simulink model "camara_termicaprofwilkley_editado_0527"  (R2022a)
settings: Solver=VariableStepAuto  StartTime=0.0  StopTime=400  RelTol=1e-3
values from neighbouring files (symbols this model uses):
  Ha = Hss.A    [Camara_Termica.m]
  Hb = Hss.B    [Camara_Termica.m]
  Hc = Hss.C    [Camara_Termica.m]
  Kcurioso = [K1 K2 K3 K4]    [Camara_Termica.m]
  Kxlinha = [Kx(:,1), Kx(:,3), Kx(:,2), Kx(:,4)]    [Camara_Termica.m]
  T = conv(T,[1 alpha])    [Camara_Termica.m]
settings Model: Creator=CARLOS HOLANDA  LastModifiedBy=CARLOS HOLANDA
settings DebuggingCC: UnconnectedInputMsg=warning  UnconnectedOutputMsg=warning  UnconnectedLineMsg=warning
settings RTWCC: DLArmComputeVersion=19.05

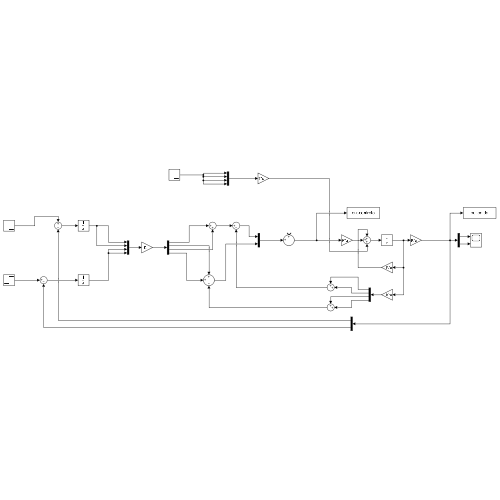
[thumbnail: Simulink's stored preview of the top-level diagram]
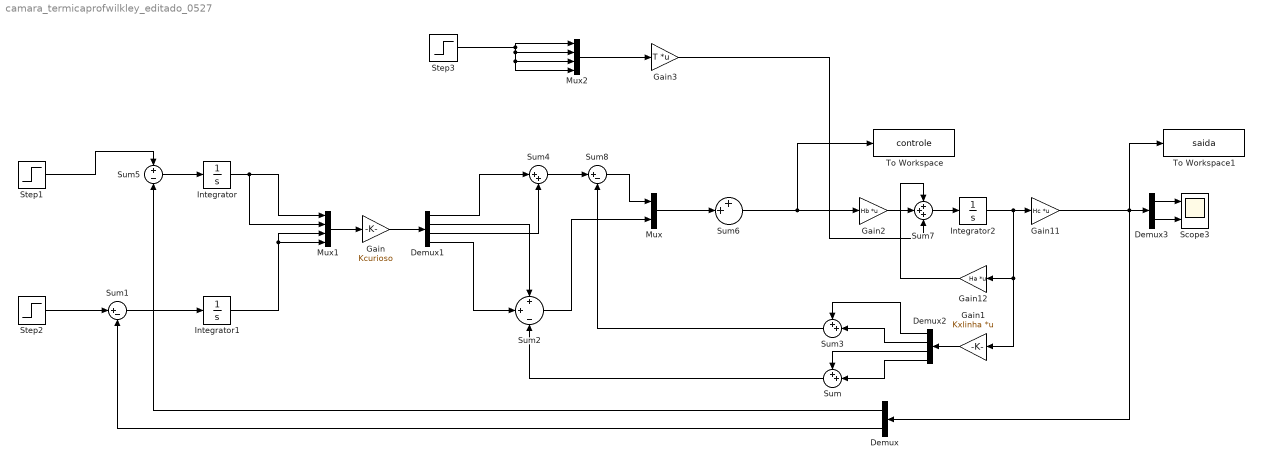
== system camara_termicaprofwilkley_editado_0527 ==
  Demux : Demux  Outputs=2
  Demux1 : Demux
  Demux2 : Demux
  Demux3 : Demux  Outputs=2
  Gain : Gain  Gain=Kcurioso
  Gain1 : Gain  Gain=Kxlinha  Multiplication=Matrix(K*u)
  Gain11 : Gain  Gain=Hc  Multiplication=Matrix(K*u)
  Gain12 : Gain  Gain=Ha  Multiplication=Matrix(K*u)
  Gain2 : Gain  Gain=Hb  Multiplication=Matrix(K*u)
  Gain3 : Gain  Gain=T  Multiplication=Matrix(K*u)
  Integrator : Integrator
  Integrator1 : Integrator
  Integrator2 : Integrator
  Mux : Mux  Inputs=2
  Mux1 : Mux
  Mux2 : Mux
  Scope3 : Scope  NumInputPorts=2
  Step1 : Step  Time=0  After=-3  SampleTime=0
  Step2 : Step  Time=100  After=2  SampleTime=0
  Step3 : Step  Time=200  After=-3  SampleTime=0
  Sum : Sum  Inputs=++|
  Sum1 : Sum  Inputs=|+-
  Sum2 : Sum  Inputs=+|+|-
  Sum3 : Sum  Inputs=++|
  Sum4 : Sum  Inputs=|++
  Sum5 : Sum  Inputs=+-
  Sum6 : Sum  Inputs=++|
  Sum7 : Sum  Inputs=+++
  Sum8 : Sum  Inputs=|+-
  To Workspace : ToWorkspace  VariableName=controle  SaveFormat=Timeseries  SampleTime=-1
  To Workspace1 : ToWorkspace  VariableName=saida  SaveFormat=Timeseries  SampleTime=-1
  wires:
  Demux3/1 -> Scope3/1
  Gain12/1 -> Sum7/2
  Sum7/1 -> Integrator2/1
  Demux3/2 -> Scope3/2
  Gain2/1 -> Sum7/1
  Demux/2 -> Sum1/2
  Step2/1 -> Sum1/1
  Sum1/1 -> Integrator1/1
  Sum8/1 -> Mux/1
  Sum2/1 -> Mux/2
  Sum3/1 -> Sum8/2
  Sum/1 -> Sum2/3
  Sum4/1 -> Sum8/1
  Integrator/1 -> Mux1/2, Mux1/1
  Mux1/1 -> Gain/1
  Gain/1 -> Demux1/1
  Demux1/1 -> Sum4/1
  Demux1/4 -> Sum2/2
  Demux1/3 -> Sum4/2
  Demux1/2 -> Sum2/1
  Integrator1/1 -> Mux1/4, Mux1/3
  Integrator2/1 -> Gain1/1, Gain12/1, Gain11/1
  Gain1/1 -> Demux2/1
  Demux2/1 -> Sum3/1
  Demux2/2 -> Sum3/2
  Demux2/3 -> Sum/1
  Demux2/4 -> Sum/2
  Gain11/1 -> To Workspace1/1, Demux/1, Demux3/1
  Sum5/1 -> Integrator/1
  Mux/1 -> Sum6/2
  Sum6/1 -> To Workspace/1, Gain2/1
  Mux2/1 -> Gain3/1
  Step3/1 -> Mux2/4, Mux2/3, Mux2/2, Mux2/1
  Demux/1 -> Sum5/2
  Step1/1 -> Sum5/1
  Gain3/1 -> Sum7/3
